simulink model "TP_MCA_QTP_2024b"  (R2024b)
settings: Solver=ode4  StartTime=0.0  StopTime=1000  FixedStep=1e-3  RelTol=1e-3
values from neighbouring files (symbols this model uses):
  MPC = struct()    [Parameters.m]
  QTP = {}    [Parameters.m]
  xref = opti.parameter(obj.nx, 1)    [MPC_controller.m]    (also in Parameters.m = [href; sol(1:2)])
settings Model: Creator=yuqi  LastModifiedBy=flo
settings ConfigComp: CovBoundaryAbsTol=1.0e-5

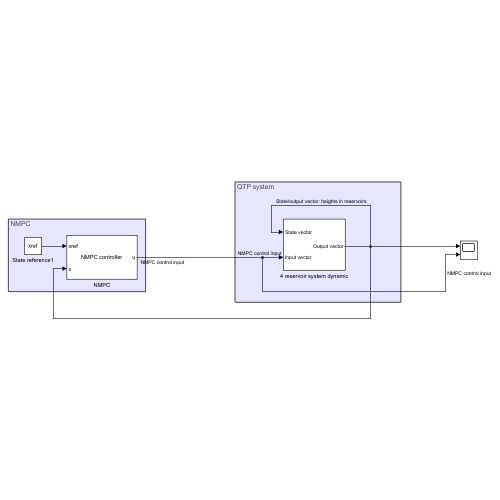
[thumbnail: Simulink's stored preview of the top-level diagram]
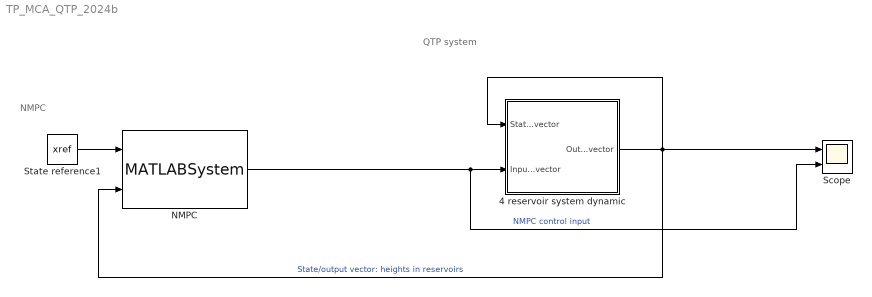
== system TP_MCA_QTP_2024b ==
  note: NMPC
  note: QTP system
  4 reservoir system dynamic : Subsystem
  NMPC : MATLABSystem  System=MPC_controller  model=MPC.model  N=MPC.N  Q=MPC.Q  R=MPC.R  P=MPC.P  xmin=MPC.xmin  xmax=MPC.xmax  umin=MPC.umin  umax=MPC.umax  dt=MPC.dt  nx=MPC.nx  nu=MPC.nu  SimulateUsing=Interpreted execution
      mask Type: MPC_controller
      mask Display:
      | disp('NMPC controller');
      | port_label('input',1,'xref');
      | port_label('input',2,'x');
      | port_label('output',1,'u');
  Scope : Scope  NumInputPorts=2
  State reference1 : Constant  Value=xref
  wires:
  4 reservoir system dynamic/1(Output vector) -> NMPC/2, Scope/1, 4 reservoir system dynamic/1(State vector)  "State/output vector: heights in reservoirs"
  State reference1/1 -> NMPC/1
  NMPC/1 -> Scope/2, 4 reservoir system dynamic/2(Input vector)  "NMPC control input"

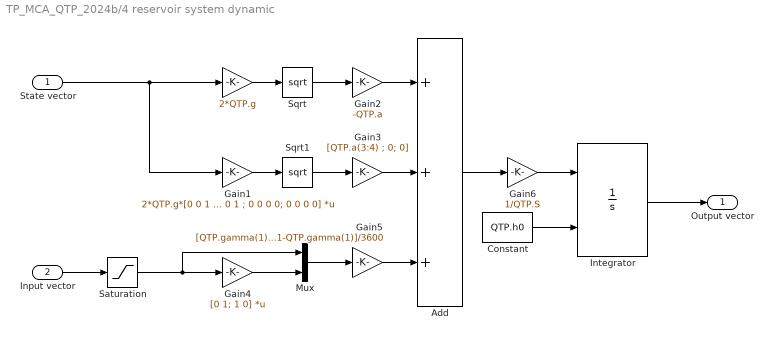
== system TP_MCA_QTP_2024b/4 reservoir system dynamic ==
  State vector : Inport
  Input vector : Inport  Port=2
  " " : Gain  Gain=2*QTP.g
  Add : Sum  Inputs=+++
  Constant : Constant  Value=QTP.h0
  Gain1 : Gain  Gain=2*QTP.g*[0 0 1 0; 0 0 0 1 ; 0 0 0 0; 0 0 0 0]  Multiplication=Matrix(K*u)
  Gain2 : Gain  Gain=-QTP.a
  Gain3 : Gain  Gain=[QTP.a(3:4) ; 0; 0]
  Gain4 : Gain  Gain=[0 1; 1 0]  Multiplication=Matrix(K*u)
  Gain5 : Gain  Gain=[QTP.gamma(1);QTP.gamma(2);1-QTP.gamma(2);1-QTP.gamma(1)]/3600
  Gain6 : Gain  Gain=1/QTP.S
  Integrator : Integrator  InitialConditionSource=external  LimitOutput=on  UpperSaturationLimit=QTP.hmax  LowerSaturationLimit=QTP.hmin
  Mux : Mux  Inputs=2
  Saturation : Saturate  UpperLimit=QTP.qmax  LowerLimit=QTP.qmin
  Sqrt : Sqrt
  Sqrt1 : Sqrt
  Output vector : Outport
  wires:
  Input vector/1 -> Saturation/1
  State vector/1 -> Gain1/1, " "/1
  Gain6/1 -> Integrator/1
  " "/1 -> Sqrt/1
  Gain1/1 -> Sqrt1/1
  Sqrt/1 -> Gain2/1
  Sqrt1/1 -> Gain3/1
  Gain2/1 -> Add/1
  Gain3/1 -> Add/2
  Gain4/1 -> Mux/2
  Mux/1 -> Gain5/1
  Gain5/1 -> Add/3
  Add/1 -> Gain6/1
  Integrator/1 -> Output vector/1
  Constant/1 -> Integrator/2
  Saturation/1 -> Mux/1, Gain4/1
